simulink model "kalman2"  (R2015b)
settings: Solver=ode45  StartTime=0.0  StopTime=500  RelTol=1e-3
values from neighbouring files (symbols this model uses):
  a = -0.02    [box1.m]    (also in kal1.mat)
  b = 1.351*10^(-3)    (= 0.001351)    [box1.m]    (also in kal1.mat)
  Ev2 = 0.0    (= 0)    [box1.m]    (also in kal1.mat)
  Ew2 = 0.7    [box1.m]    (also in kal1.mat)
  l = 0.980    (= 0.98)    [box1.m]    (also in kal1.mat)
settings Model: Creator=ry0  LastModifiedBy=inoma-ubu
settings DataIOCC: SaveFormat=Array
settings HardwareCC: ProdBitPerPointer=32  ProdLargestAtomicFloat=None  ProdIntDivRoundTo=Undefined  ProdEndianess=Unspecified  ProdWordSize=32  ProdHWDeviceType=32-bit Generic
settings GRTTargetCC: GeneratePreprocessorConditionals=Disable all
settings ConfigComp: CovModelRefEnable=Off

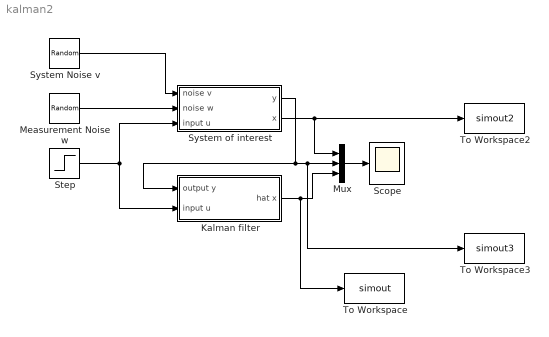
== system kalman2 ==
  Kalman filter : Subsystem
  Measurement Noise w : RandomNumber  Variance=Ew2  Seed=8  SampleTime=0.1
  Mux : Mux  Inputs=3
  Scope : Scope
  Step : Step  After=500  SampleTime=0
  System Noise v : RandomNumber  Variance=Ev2  Seed=5  SampleTime=0.1
  System of interest : Subsystem
  To Workspace : ToWorkspace  VariableName=simout  SaveFormat=Structure With Time  SampleTime=-1
  "To Workspace2 " : ToWorkspace  VariableName=simout2  SaveFormat=Structure With Time  SampleTime=-1
  To Workspace3 : ToWorkspace  VariableName=simout3  SaveFormat=Structure With Time  SampleTime=-1
  wires:
  Measurement Noise w/1 -> System of interest/2(noise w)
  System Noise v/1 -> System of interest/1(noise v)
  Step/1 -> Kalman filter/2("input u "), System of interest/3("input u ")
  Mux/1 -> Scope/1
  System of interest/2(x) -> "To Workspace2 "/1, Mux/1
  Kalman filter/1(hat x) -> To Workspace/1, Mux/3
  System of interest/1(y) -> To Workspace3/1, Mux/2, Kalman filter/1(output y)

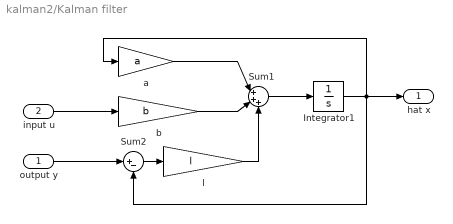
== system kalman2/Kalman filter ==
  output y : Inport
  "input u " : Inport  Port=2
  Integrator1 : Integrator
  Sum1 : Sum  Inputs=|+++
  Sum2 : Sum  Inputs=|+-
  a : Gain  Gain=a
  b : Gain  Gain=b
  l : Gain  Gain=l
  hat x : Outport
  wires:
  output y/1 -> Sum2/1
  "input u "/1 -> b/1
  Sum1/1 -> Integrator1/1
  Integrator1/1 -> a/1, Sum2/2, hat x/1
  Sum2/1 -> l/1
  a/1 -> Sum1/1
  b/1 -> Sum1/2
  l/1 -> Sum1/3

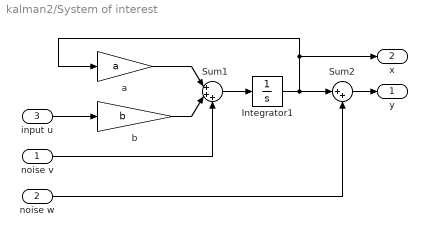
== system kalman2/System of interest ==
  noise v : Inport
  noise w : Inport  Port=2
  "input u " : Inport  Port=3
  Integrator1 : Integrator
  Sum1 : Sum  Inputs=|+++
  Sum2 : Sum  Inputs=|++
  a : Gain  Gain=a
  b : Gain  Gain=b
  y : Outport
  x : Outport  Port=2
  wires:
  noise v/1 -> Sum1/3
  Sum2/1 -> y/1
  noise w/1 -> Sum2/2
  "input u "/1 -> b/1
  Sum1/1 -> Integrator1/1
  Integrator1/1 -> Sum2/1, x/1, a/1
  a/1 -> Sum1/1
  b/1 -> Sum1/2
